simulink model "NUbotsUDPTest"  (R2019b)
settings: Solver=VariableStepAuto  StartTime=0.0  StopTime=10.0  RelTol=1e-3
libraries: NUbotsUDP x2, dspnetwork x1
settings Model: Creator=cameron  LastModifiedBy=cameron

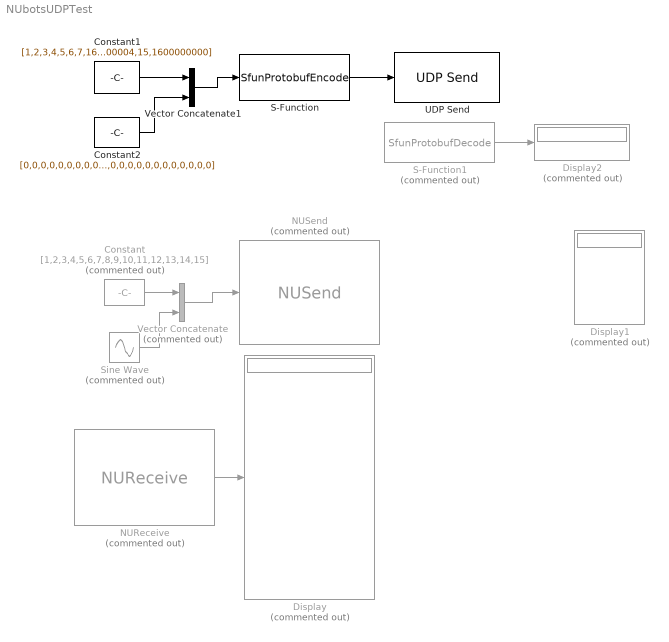
== system NUbotsUDPTest ==
  Constant : Constant  Commented=on  Value=[1,2,3,4,5,6,7,8,9,10,11,12,13,14,15]  OutDataTypeStr=double  SampleTime=0.1
  Constant1 : Constant  Value=[1,2,3,4,5,6,7,160,9,10,11,12,13,100004,15,1600000000]  OutDataTypeStr=double  SampleTime=0.1
  Constant2 : Constant  Value=[0,0,0,0,0,0,0,0,0,0,0,0,0,0,0,0,0,0,0,0,0,0,0,0,0,0,0,0,0,0,0,0,0,0,0,0,0,0,0,0,0,0,0,0,0,0,0,0,0,0,0,0,0,0,0,0,0,0,0,0,0,0,0,0,0,0,0,0,0,0,0,0,0,0,0,0,0,0,0,0,0,0,0,0,0,0,0,0,0,0,0,0,0,0,0,0,0,0,0,0,0,0,0,0,0,0,0,0,0,0,0,0,0,0,0,0,0,0,0,0,0,0,0,0,0,0,0,0,0,0,0,0,0,0,0,0,0,0,0,0,0,0,0,0,0,0,0,0,0,0,0,0,0,0,0,0,0,0,0,0,0,0,0,0,0,0,0,0,0,0,0,0,0,0,0,0,0,0,0,0,0,0,0,0,0,0,0,0,0,0,0,0,0,0,0,0,0,0,0,0,0,0,0,0,0,0,0,0,0,0,0,0,0,0,0,0,0,0,0,0,0,0,0,0,0,0,0,0,0,0,0,0,0,0,0,0,0,0,0,0]
  Display : Display  Commented=on
      settings: Format=long_e
  Display1 : Display  Commented=on
  Display2 : Display  Commented=on
  NUReceive : NUbotsUDP/NUReceive  Commented=on  LocalPort=5002  RemotePort=5001
  NUSend : NUbotsUDP/NUSend  Commented=on  LocalPort=5001  RemotePort=5002
  S-Function : S-Function  FunctionName=SfunProtobufEncode  SFunctionDeploymentMode=off  EnableBusSupport=off
  S-Function1 : S-Function  Commented=on  FunctionName=SfunProtobufDecode  SFunctionDeploymentMode=off  EnableBusSupport=off
  Sine Wave : Sin  Commented=on  SampleTime=0.1
  UDP Send : dspnetwork/UDP Send  remoteURL='127.0.0.1'  remotePort=25000  localURL='0.0.0.0'  localPortSource=Automatically determine  localPort=-1  sampletime=-1  blockPlatform=[]  separateLengthPort=0
      settings: SourceProductName=Simulink
  Vector Concatenate : Concatenate  Commented=on
  Vector Concatenate1 : Concatenate
  wires:
  NUReceive/1 -> Display/1
  Constant/1 -> Vector Concatenate/1
  Vector Concatenate/1 -> NUSend/1
  Sine Wave/1 -> Vector Concatenate/2
  Constant2/1 -> Vector Concatenate1/2
  S-Function1/1 -> Display2/1
  Constant1/1 -> Vector Concatenate1/1
  Vector Concatenate1/1 -> S-Function/1
  S-Function/1 -> UDP Send/1
